simulink model "python_calibration_exec"  (Simulink 3.00)
libraries: execlib x5
settings Model: MaskType=REX sequence  MaskIconFrame=on  MaskIconOpaque=on  MaskIconRotate=none  MaskIconUnits=autoscale

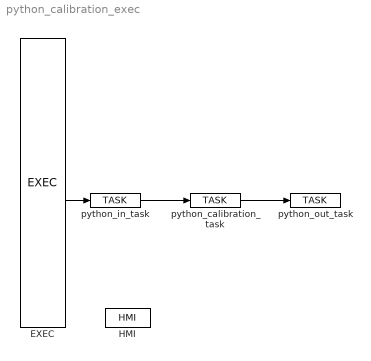
== system python_calibration_exec ==
  EXEC : execlib/EXEC  target=Generic target device  tick=0.005  ntick0=10  ntick1=20  ntick2=100  ntick3=1200  pri0=5  pri1=9  pri2=13  pri3=18  cpu0=-1  cpu1=-1  cpu2=-1  cpu3=-1
  HMI : execlib/HMI  IncludeHMI=on  HmiDir=hmi  SourceDir=hmisrc  GenerateWebWatch=off  GenerateRexHMI=on  RedirectToHMI=on  Compression=on
  python_calibration_task : execlib/TASK  factor=1  start=2  stop=3  stack=10240  MDLOPEN=on
  python_in_task : execlib/TASK  factor=1  start=1  stop=2  stack=10240  MDLOPEN=on
  python_out_task : execlib/TASK  factor=1  start=3  stop=4  stack=10240  MDLOPEN=on
  wires:
  EXEC/5 -> python_in_task/1
  python_calibration_task/1 -> python_out_task/1
  python_in_task/1 -> python_calibration_task/1
